simulink model "ASM_sim"  (R2020a)
settings: Solver=ode1  StartTime=0.0  StopTime=70  FixedStep=0.001  RelTol=1e-3
undefined symbols (not defined in the file or in its folder): kd, kp
settings Model: Creator=yshang  LastModifiedBy=jerry
settings DataIOCC: ReturnWorkspaceOutputs=off
settings DebuggingCC: ArithmeticOperatorsInVariantConditions=warning
settings SFSimCC: SimUseLocalCustomCode=off  CustomCodeUndefinedFunction=UseInterfaceOnly
settings RTWCC: RTWUseLocalCustomCode=off
settings CodeAppCC: StateflowObjectComments=on

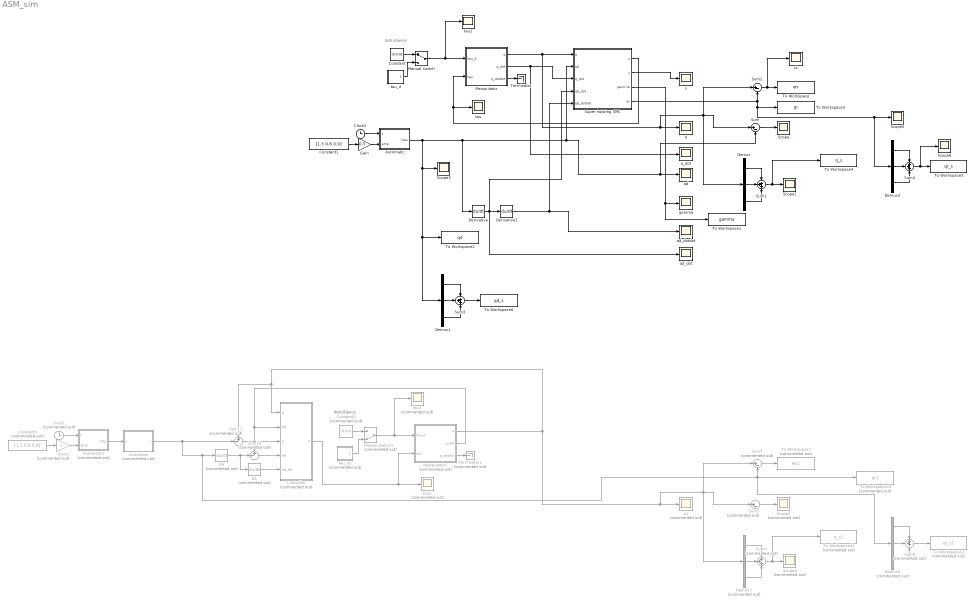
== system ASM_sim ==
  note: disturbance
  note: disturbance
  Automatic : MATLAB Function  TreatAsAtomicUnit=on
  Automatic1 : MATLAB Function  Commented=on  TreatAsAtomicUnit=on
  Clock1 : Clock  Commented=on
  Clock2 : Clock
  Constant : Constant  Value=[0;0;0]
  Constant1 : Constant  Value=[1.5 0.6 0.9]'  SampleTime=0.001
  Constant2 : Constant  Commented=on  Value=[0;0;0]
  Constant3 : Constant  Commented=on  Value=[1.5 0.6 0.9]'  SampleTime=0.001
  Controller : Subsystem  Commented=on
  D4 : Derivative  Commented=on
  D5 : Derivative  Commented=on
  Demux : Demux  Outputs=3
  Demux1 : Demux  Outputs=3
  Demux2 : Demux  Outputs=3
  Demux3 : Demux  Commented=on  Outputs=3
  Demux5 : Demux  Commented=on  Outputs=3
  Derivative : Derivative
  Derivative1 : Derivative
  Gain : Gain  Gain=0.5
  Gain1 : Gain  Commented=on
  Invariance : MATLAB Function  Commented=on  TreatAsAtomicUnit=on
  Manipulator : Subsystem
  Manipulator1 : Subsystem  Commented=on
  Manual Switch : ManualSwitch
  Manual Switch1 : ManualSwitch  Commented=on  CurrentSetting=0
  Scope{,1,3,5..6} (5 alike) : Scope
  Scope2 : Scope  Commented=on
  Scope4 : Scope  Commented=on
  Sum : Sum  Inputs=|+-
  Sum1 : Sum  Inputs=+++
  Sum10 : Sum  Commented=on  Inputs=+-|
  Sum11 : Sum  Commented=on  Inputs=+-|
  Sum2 : Sum  Inputs=|+-
  Sum3 : Sum  Inputs=+++
  Sum4 : Sum  Inputs=+++
  Sum5 : Sum  Commented=on  Inputs=|+-
  Sum6 : Sum  Commented=on  Inputs=+++
  Sum7 : Sum  Commented=on  Inputs=|+-
  Sum9 : Sum  Commented=on  Inputs=+++
  Super twisting SMC : Subsystem
  Terminator : Terminator
  Terminator1 : Terminator  Commented=on
  To Workspace : ToWorkspace  VariableName=err  SampleTime=0.001
  To Workspace1 : ToWorkspace  VariableName=gamma  SampleTime=0.001
  To Workspace10 : ToWorkspace  Commented=on  VariableName=qr1  SampleTime=0.001
  To Workspace11 : ToWorkspace  Commented=on  VariableName=q_s1  SampleTime=0.001
  To Workspace12 : ToWorkspace  Commented=on  VariableName=qr_s1  SampleTime=0.001
  To Workspace2 : ToWorkspace  VariableName=qd  SampleTime=0.001
  To Workspace3 : ToWorkspace  VariableName=qr  SampleTime=0.001
  To Workspace4 : ToWorkspace  VariableName=q_s  SampleTime=0.001
  To Workspace5 : ToWorkspace  VariableName=qr_s  SampleTime=0.001
  To Workspace6 : ToWorkspace  VariableName=qd_s  SampleTime=0.001
  To Workspace7 : ToWorkspace  Commented=on  VariableName=err1  SampleTime=0.001
  gamma : Scope
  q : Scope
  q1 : Scope  Commented=on
  q_dot : Scope
  qd : Scope
  qd_dot : Scope
  qd_dotdot : Scope
  s : Scope
  s1 : Scope
  tau : Scope
  tau1 : Scope
  tau2 : Scope  Commented=on
  tau3 : Scope  Commented=on
  tau_d : Subsystem
  tau_d1 : Subsystem  Commented=on
  wires:
  Manual Switch/1 -> tau1/1, Manipulator/1(tau_d)
  Constant/1 -> Manual Switch/1
  Manipulator/1(q) -> Super twisting SMC/1(q), Sum2/1, Demux/1, Sum/1, q/1
  Manipulator/2(q_dot) -> Super twisting SMC/3(q_dot), q_dot/1
  Super twisting SMC/1(u) -> Manipulator/2(tau), tau/1
  tau_d/1(tau_dist) -> Manual Switch/2
  Super twisting SMC/2(s) -> s/1
  Super twisting SMC/3(gamma) -> To Workspace1/1, gamma/1
  Derivative/1 -> Super twisting SMC/4(qd_dot), qd_dot/1, Derivative1/1
  Manipulator/3(q_dotdot) -> Terminator/1
  Derivative1/1 -> Super twisting SMC/5(qd_dotdot), qd_dotdot/1
  Sum/1 -> Scope/1
  Demux/2 -> Sum1/2
  Demux/1 -> Sum1/1
  Demux/3 -> Sum1/3
  Sum1/1 -> To Workspace4/1, Scope1/1
  Constant1/1 -> Gain/1
  Clock2/1 -> Automatic/1(t)
  Gain/1 -> Automatic/2(amp)
  Sum2/1 -> s1/1, To Workspace/1
  Demux1/2 -> Sum3/2
  Demux1/1 -> Sum3/1
  Automatic/1(Des) -> Demux1/1, To Workspace2/1, Scope3/1, Derivative/1, Super twisting SMC/2(qd), Sum/2, qd/1
  Sum3/1 -> To Workspace6/1
  Demux1/3 -> Sum3/3
  Demux2/2 -> Sum4/2
  Demux2/1 -> Sum4/1
  Super twisting SMC/4(qr) -> Scope5/1, Demux2/1, To Workspace3/1, Sum2/2
  Sum4/1 -> Scope6/1, To Workspace5/1
  Demux2/3 -> Sum4/3
  Sum7/1 -> To Workspace7/1
  Sum6/1 -> To Workspace11/1, Scope4/1
  Demux5/3 -> Sum9/3
  Demux3/1 -> Sum6/1
  Constant2/1 -> Manual Switch1/1
  Invariance/1(y) -> Demux5/1, To Workspace10/1, Sum7/2, D4/1, Sum11/2
  tau_d1/1(tau_dist) -> Manual Switch1/2
  Sum5/1 -> Scope2/1
  Manipulator1/3(q_dotdot) -> Terminator1/1
  Demux5/2 -> Sum9/2
  Controller/1(T) -> Manipulator1/2(tau), tau2/1
  Manual Switch1/1 -> tau3/1, Manipulator1/1(tau_d)
  Demux3/3 -> Sum6/3
  Demux3/2 -> Sum6/2
  Demux5/1 -> Sum9/1
  Sum9/1 -> To Workspace12/1
  Gain1/1 -> Automatic1/2(amp)
  Clock1/1 -> Automatic1/1(t)
  Constant3/1 -> Gain1/1
  Automatic1/1(Des) -> Invariance/1(u)
  Sum11/1 -> Controller/3(e)
  Manipulator1/2(q_dot) -> Controller/2(qd), Sum10/1
  Manipulator1/1(q) -> Sum11/1, Controller/1(q), Sum7/1, Demux3/1, Sum5/1, q1/1
  D4/1 -> D5/1, Sum10/2
  D5/1 -> Controller/5(qd_dd)
  Sum10/1 -> Controller/4(ed)

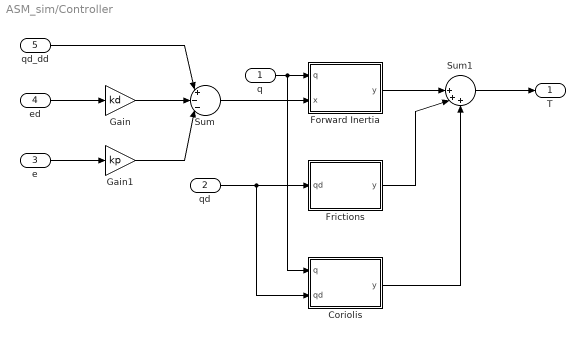
== system ASM_sim/Controller ==
  q : Inport
  qd : Inport  Port=2
  e : Inport  Port=3
  ed : Inport  Port=4
  qd_dd : Inport  Port=5
  Coriolis : MATLAB Function  TreatAsAtomicUnit=on
  Forward Inertia : MATLAB Function  TreatAsAtomicUnit=on
  Frictions : MATLAB Function  TreatAsAtomicUnit=on
  Gain : Gain  Gain=kd
  Gain1 : Gain  Gain=kp
  Sum : Sum  Inputs=|+--|
  Sum1 : Sum  Inputs=||+++
  T : Outport
  wires:
  q/1 -> Coriolis/1(q), Forward Inertia/1(q)
  qd_dd/1 -> Sum/1
  ed/1 -> Gain/1
  Gain/1 -> Sum/2
  e/1 -> Gain1/1
  Gain1/1 -> Sum/3
  Sum/1 -> Forward Inertia/2(x)
  qd/1 -> Coriolis/2(qd), Frictions/1(qd)
  Forward Inertia/1(y) -> Sum1/1
  Frictions/1(y) -> Sum1/2
  Sum1/1 -> T/1
  Coriolis/1(y) -> Sum1/3

== system ASM_sim/Manipulator ==
  tau_d : Inport
  tau : Inport  Port=2
  Integrator : Integrator  InitialCondition=[0;0;0]  ContinuousStateAttributes='velocity'
  Integrator1 : Integrator  InitialCondition=[0;0;0]  ContinuousStateAttributes='position'
  Robot : MATLAB Function  TreatAsAtomicUnit=on
  Sum : Sum  Inputs=|++
  q : Outport  VectorParamsAs1DForOutWhenUnconnected=off
  q_dot : Outport  Port=2  VectorParamsAs1DForOutWhenUnconnected=off
  q_dotdot : Outport  Port=3  VectorParamsAs1DForOutWhenUnconnected=off
  wires:
  Integrator1/1 -> Robot/2(q), q/1
  Robot/1(qdd) -> q_dotdot/1, Integrator/1
  Integrator/1 -> q_dot/1, Robot/3(qd), Integrator1/1
  Sum/1 -> Robot/1(T)
  tau_d/1 -> Sum/1
  tau/1 -> Sum/2

== system ASM_sim/Manipulator1 ==
  tau_d : Inport
  tau : Inport  Port=2
  Integrator : Integrator  InitialCondition=[0;0;0]  ContinuousStateAttributes='velocity'
  Integrator1 : Integrator  InitialCondition=[0;0;0]  ContinuousStateAttributes='position'
  Robot : MATLAB Function  TreatAsAtomicUnit=on
  Sum : Sum  Inputs=|++
  q : Outport  VectorParamsAs1DForOutWhenUnconnected=off
  q_dot : Outport  Port=2  VectorParamsAs1DForOutWhenUnconnected=off
  q_dotdot : Outport  Port=3  VectorParamsAs1DForOutWhenUnconnected=off
  wires:
  Integrator1/1 -> Robot/2(q), q/1
  Robot/1(qdd) -> q_dotdot/1, Integrator/1
  Integrator/1 -> q_dot/1, Robot/3(qd), Integrator1/1
  Sum/1 -> Robot/1(T)
  tau_d/1 -> Sum/1
  tau/1 -> Sum/2

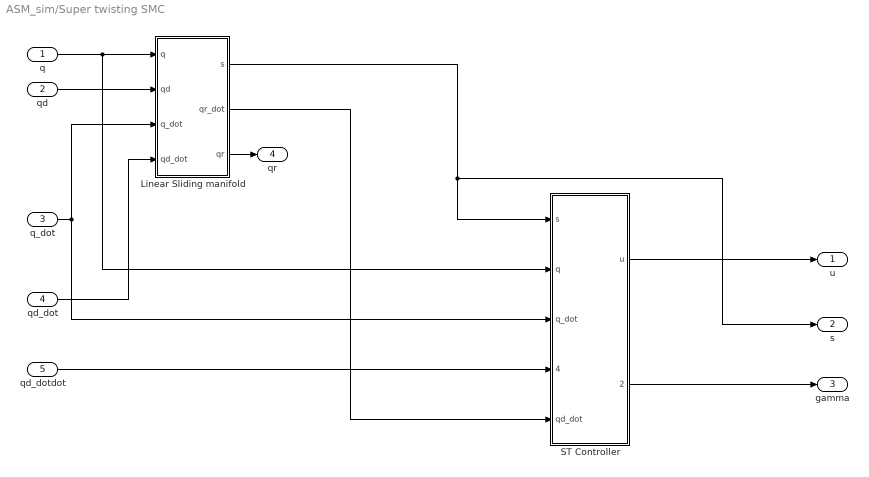
== system ASM_sim/Super twisting SMC ==
  q : Inport
  qd : Inport  Port=2
  q_dot : Inport  Port=3
  qd_dot : Inport  Port=4
  qd_dotdot : Inport  Port=5
  Linear Sliding manifold : Subsystem
  ST Controller : Subsystem
  u : Outport  VectorParamsAs1DForOutWhenUnconnected=off
  s : Outport  Port=2  VectorParamsAs1DForOutWhenUnconnected=off
  gamma : Outport  Port=3  VectorParamsAs1DForOutWhenUnconnected=off
  qr : Outport  Port=4  VectorParamsAs1DForOutWhenUnconnected=off
  wires:
  q/1 -> Linear Sliding manifold/1(q), ST Controller/2(q)
  q_dot/1 -> Linear Sliding manifold/3(q_dot), ST Controller/3(q_dot)
  Linear Sliding manifold/1(s) -> s/1, ST Controller/1(s)
  qd/1 -> Linear Sliding manifold/2(qd)
  ST Controller/1(u) -> u/1
  ST Controller/2(gamma) -> gamma/1
  qd_dot/1 -> Linear Sliding manifold/4(qd_dot)
  qd_dotdot/1 -> ST Controller/4(qd_dotdot)
  Linear Sliding manifold/2(qr_dot) -> ST Controller/5("qd_dot ")
  Linear Sliding manifold/3(qr) -> qr/1

== system ASM_sim/tau_d ==
  Mux1 : Mux  Inputs=3
  Sine Wave3 : Sin  Amplitude=0.3  Frequency=2  SampleTime=0
  Sine Wave4 : Sin  Amplitude=0.2  Frequency=4  SampleTime=0
  Sine Wave5 : Sin  Amplitude=0.1  Frequency=3  SampleTime=0
  tau_dist : Outport  VectorParamsAs1DForOutWhenUnconnected=off
  wires:
  Sine Wave4/1 -> Mux1/2
  Mux1/1 -> tau_dist/1
  Sine Wave3/1 -> Mux1/1
  Sine Wave5/1 -> Mux1/3

== system ASM_sim/tau_d1 ==
  Mux1 : Mux  Inputs=3
  Sine Wave3 : Sin  Amplitude=0.3  Frequency=2  SampleTime=0
  Sine Wave4 : Sin  Amplitude=0.2  Frequency=4  SampleTime=0
  Sine Wave5 : Sin  Amplitude=0.1  Frequency=3  SampleTime=0
  tau_dist : Outport  VectorParamsAs1DForOutWhenUnconnected=off
  wires:
  Sine Wave4/1 -> Mux1/2
  Mux1/1 -> tau_dist/1
  Sine Wave3/1 -> Mux1/1
  Sine Wave5/1 -> Mux1/3

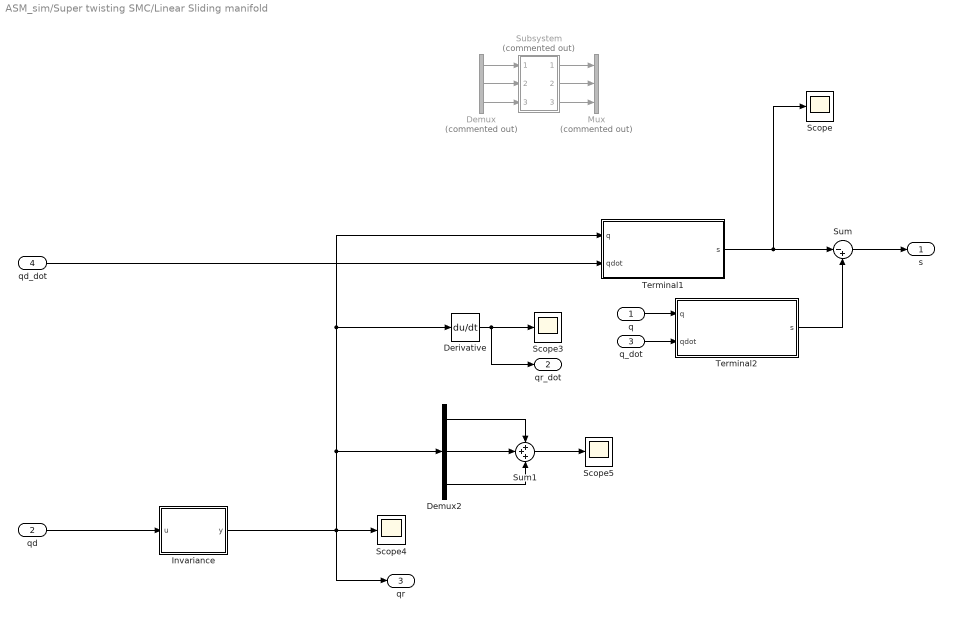
== system ASM_sim/Super twisting SMC/Linear Sliding manifold ==
  q : Inport
  qd : Inport  Port=2
  q_dot : Inport  Port=3
  qd_dot : Inport  Port=4
  Demux : Demux  Commented=on  Outputs=3
  Demux2 : Demux  Outputs=3
  Derivative : Derivative
  Invariance : MATLAB Function  TreatAsAtomicUnit=on
  Mux : Mux  Commented=on  Inputs=3
  Scope{,3..5} (4 alike) : Scope
  Subsystem : Subsystem  Commented=on
  Sum : Sum  Inputs=|-+
  Sum1 : Sum  Inputs=+++
  Terminal1 : Subsystem
  Terminal2 : Subsystem
  s : Outport  VectorParamsAs1DForOutWhenUnconnected=off
  qr_dot : Outport  Port=2  VectorParamsAs1DForOutWhenUnconnected=off
  qr : Outport  Port=3  VectorParamsAs1DForOutWhenUnconnected=off
  wires:
  q/1 -> Terminal2/1(q)
  q_dot/1 -> Terminal2/2(qdot)
  Terminal2/1(s) -> Sum/2
  Sum/1 -> s/1
  Demux2/3 -> Sum1/3
  qd/1 -> Invariance/1(u)
  Derivative/1 -> qr_dot/1, Scope3/1
  Demux2/2 -> Sum1/2
  Sum1/1 -> Scope5/1
  Demux2/1 -> Sum1/1
  Terminal1/1(s) -> Scope/1, Sum/1
  qd_dot/1 -> Terminal1/2(qdot)
  Invariance/1(y) -> qr/1, Demux2/1, Terminal1/1(q), Derivative/1, Scope4/1
  Demux/2 -> Subsystem/2(In2)
  Subsystem/3(Out3) -> Mux/3
  Demux/1 -> Subsystem/1(In1)
  Subsystem/1(Out1) -> Mux/1
  Demux/3 -> Subsystem/3(In3)
  Subsystem/2(Out2) -> Mux/2

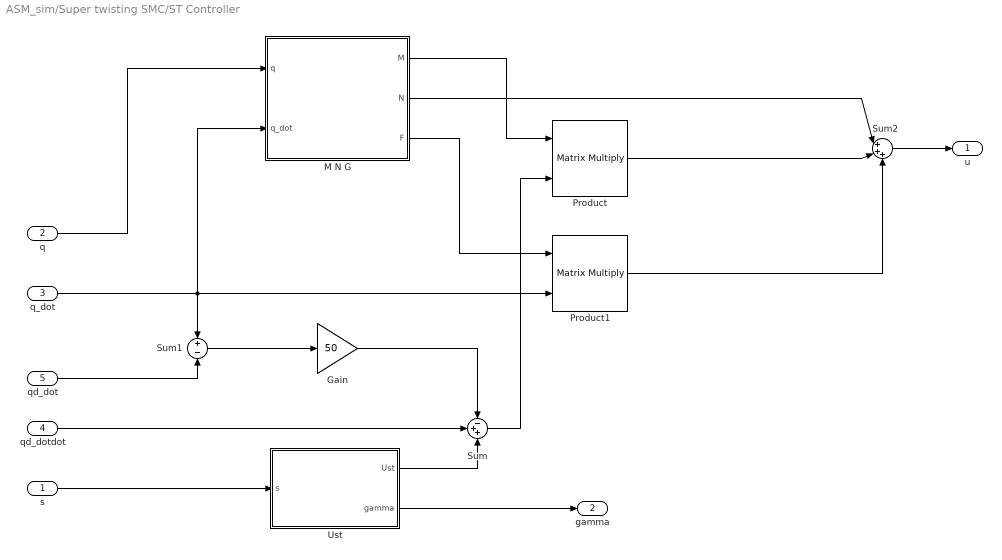
== system ASM_sim/Super twisting SMC/ST Controller ==
  s : Inport
  q : Inport  Port=2
  q_dot : Inport  Port=3
  qd_dotdot : Inport  Port=4
  "qd_dot " : Inport  Port=5
  Gain : Gain  Gain=50
  M N G : MATLAB Function  TreatAsAtomicUnit=on
  Product : Product  Multiplication=Matrix(*)
  Product1 : Product  Multiplication=Matrix(*)
  Sum : Sum  Inputs=-++
  Sum1 : Sum  Inputs=+|-
  Sum2 : Sum  Inputs=|+++
  Ust : Subsystem
  u : Outport  VectorParamsAs1DForOutWhenUnconnected=off
  gamma : Outport  Port=2  VectorParamsAs1DForOutWhenUnconnected=off
  wires:
  s/1 -> Ust/1(s)
  Ust/2(gamma) -> gamma/1
  Sum/1 -> Product/2
  Ust/1(Ust) -> Sum/3
  M N G/3(F) -> Product1/1
  M N G/1(M) -> Product/1
  q/1 -> M N G/1(q)
  q_dot/1 -> M N G/2(q_dot), Product1/2, Sum1/1
  Product1/1 -> Sum2/3
  Sum2/1 -> u/1
  "qd_dot "/1 -> Sum1/2
  Sum1/1 -> Gain/1
  qd_dotdot/1 -> Sum/2
  Gain/1 -> Sum/1
  M N G/2(N) -> Sum2/1
  Product/1 -> Sum2/2

== system ASM_sim/Super twisting SMC/Linear Sliding manifold/Subsystem ==
  In1 : Inport
  In2 : Inport  Port=2
  In3 : Inport  Port=3
  Transfer Fcn : TransferFcn  Denominator=[0.01 1]
  Transfer Fcn1 : TransferFcn  Denominator=[0.01 1]
  Transfer Fcn2 : TransferFcn  Denominator=[0.01 1]
  Out1 : Outport
  Out2 : Outport  Port=2
  Out3 : Outport  Port=3
  wires:
  Transfer Fcn/1 -> Out1/1
  Transfer Fcn1/1 -> Out2/1
  In2/1 -> Transfer Fcn1/1
  In1/1 -> Transfer Fcn/1
  Transfer Fcn2/1 -> Out3/1
  In3/1 -> Transfer Fcn2/1

== system ASM_sim/Super twisting SMC/Linear Sliding manifold/Terminal1 ==
  q : Inport
  qdot : Inport  Port=2
  Gain1 : Gain  Gain=50
  Sum5 : Sum  Inputs=|++
  s : Outport  VectorParamsAs1DForOutWhenUnconnected=off
  wires:
  q/1 -> Gain1/1
  Sum5/1 -> s/1
  Gain1/1 -> Sum5/1
  qdot/1 -> Sum5/2

== system ASM_sim/Super twisting SMC/Linear Sliding manifold/Terminal2 ==
  q : Inport
  qdot : Inport  Port=2
  Gain1 : Gain  Gain=50
  Sum5 : Sum  Inputs=|++
  s : Outport  VectorParamsAs1DForOutWhenUnconnected=off
  wires:
  q/1 -> Gain1/1
  Sum5/1 -> s/1
  Gain1/1 -> Sum5/1
  qdot/1 -> Sum5/2

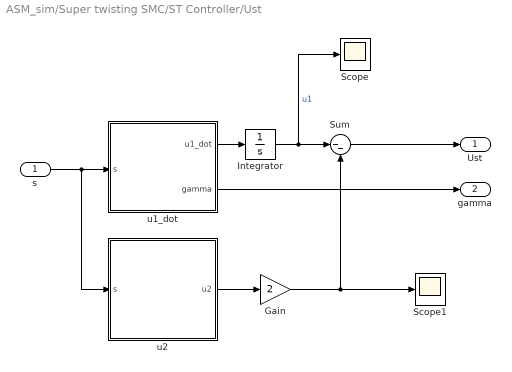
== system ASM_sim/Super twisting SMC/ST Controller/Ust ==
  s : Inport
  Gain : Gain  Gain=2
  Integrator : Integrator
  Scope : Scope
  Scope1 : Scope
  Sum : Sum  Inputs=|--
  u1_dot : Subsystem
  u2 : Subsystem
  Ust : Outport  VectorParamsAs1DForOutWhenUnconnected=off
  gamma : Outport  Port=2  VectorParamsAs1DForOutWhenUnconnected=off
  wires:
  s/1 -> u2/1(s), u1_dot/1(s)
  u1_dot/1(u1_dot) -> Integrator/1
  Integrator/1 -> Sum/1, Scope/1  "u1"
  u2/1(u2) -> Gain/1
  Sum/1 -> Ust/1
  u1_dot/2(gamma) -> gamma/1
  Gain/1 -> Scope1/1, Sum/2

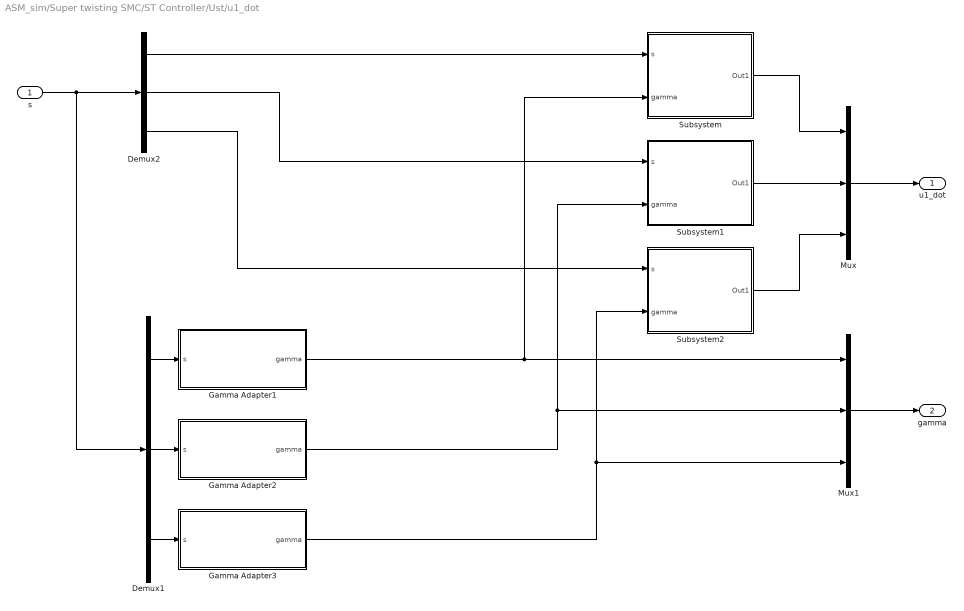
== system ASM_sim/Super twisting SMC/ST Controller/Ust/u1_dot ==
  s : Inport
  Demux1 : Demux  Outputs=3
  Demux2 : Demux  Outputs=3
  Gamma Adapter1 : Subsystem
  Gamma Adapter2 : Subsystem
  Gamma Adapter3 : Subsystem
  Mux : Mux  Inputs=3
  Mux1 : Mux  Inputs=3
  Subsystem : Subsystem
  Subsystem1 : Subsystem
  Subsystem2 : Subsystem
  u1_dot : Outport  VectorParamsAs1DForOutWhenUnconnected=off
  gamma : Outport  Port=2  VectorParamsAs1DForOutWhenUnconnected=off
  wires:
  Mux/1 -> u1_dot/1
  s/1 -> Demux1/1, Demux2/1
  Demux2/1 -> Subsystem/1(s)
  Demux2/2 -> Subsystem1/1(s)
  Subsystem1/1(Out1) -> Mux/2
  Subsystem/1(Out1) -> Mux/1
  Subsystem2/1(Out1) -> Mux/3
  Demux2/3 -> Subsystem2/1(s)
  Demux1/1 -> Gamma Adapter1/1(s)
  Demux1/3 -> Gamma Adapter3/1(s)
  Demux1/2 -> Gamma Adapter2/1(s)
  Mux1/1 -> gamma/1
  Gamma Adapter1/1(gamma) -> Subsystem/2(gamma), Mux1/1
  Gamma Adapter2/1(gamma) -> Subsystem1/2(gamma), Mux1/2
  Gamma Adapter3/1(gamma) -> Subsystem2/2(gamma), Mux1/3

== system ASM_sim/Super twisting SMC/ST Controller/Ust/u2 ==
  s : Inport
  Demux : Demux  Outputs=3
  Mux : Mux  Inputs=3
  Subsystem : Subsystem
  Subsystem1 : Subsystem
  Subsystem3 : Subsystem
  u2 : Outport  VectorParamsAs1DForOutWhenUnconnected=off
  wires:
  Mux/1 -> u2/1
  s/1 -> Demux/1
  Demux/1 -> Subsystem/1(In1)
  Subsystem/1(Out1) -> Mux/1
  Demux/3 -> Subsystem3/1(In1)
  Demux/2 -> Subsystem1/1(In1)
  Subsystem1/1(Out1) -> Mux/2
  Subsystem3/1(Out1) -> Mux/3

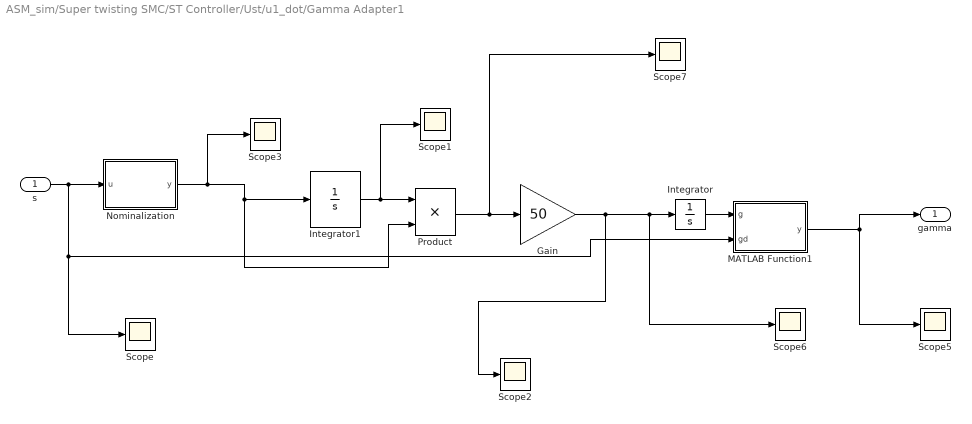
== system ASM_sim/Super twisting SMC/ST Controller/Ust/u1_dot/Gamma Adapter1 ==
  s : Inport
  Gain : Gain  Gain=50
  Integrator : Integrator
  Integrator1 : Integrator
  MATLAB Function1 : MATLAB Function  TreatAsAtomicUnit=on
  Nominalization : MATLAB Function  TreatAsAtomicUnit=on
  Product : Product
  Scope{,1..3,5..7} (7 alike) : Scope
  gamma : Outport  VectorParamsAs1DForOutWhenUnconnected=off
  wires:
  MATLAB Function1/1(y) -> gamma/1, Scope5/1
  Integrator1/1 -> Product/1, Scope1/1
  s/1 -> Scope/1, MATLAB Function1/2(gd), Nominalization/1(u)
  Nominalization/1(y) -> Integrator1/1, Product/2, Scope3/1
  Product/1 -> Gain/1, Scope7/1
  Gain/1 -> Scope6/1, Integrator/1, Scope2/1
  Integrator/1 -> MATLAB Function1/1(g)

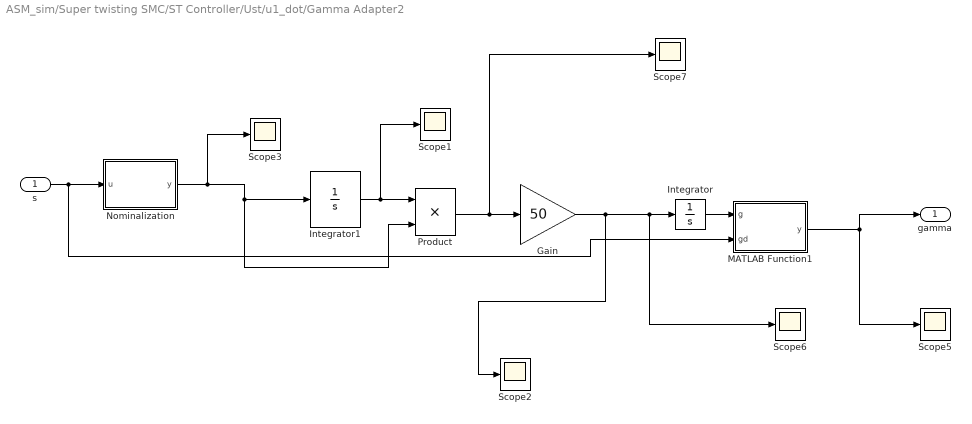
== system ASM_sim/Super twisting SMC/ST Controller/Ust/u1_dot/Gamma Adapter2 ==
  s : Inport
  Gain : Gain  Gain=50
  Integrator : Integrator
  Integrator1 : Integrator
  MATLAB Function1 : MATLAB Function  TreatAsAtomicUnit=on
  Nominalization : MATLAB Function  TreatAsAtomicUnit=on
  Product : Product
  Scope{1..3,5..7} (6 alike) : Scope
  gamma : Outport  VectorParamsAs1DForOutWhenUnconnected=off
  wires:
  Integrator/1 -> MATLAB Function1/1(g)
  Gain/1 -> Scope2/1, Integrator/1, Scope6/1
  Product/1 -> Scope7/1, Gain/1
  Nominalization/1(y) -> Scope3/1, Product/2, Integrator1/1
  s/1 -> Nominalization/1(u), MATLAB Function1/2(gd)
  Integrator1/1 -> Scope1/1, Product/1
  MATLAB Function1/1(y) -> Scope5/1, gamma/1

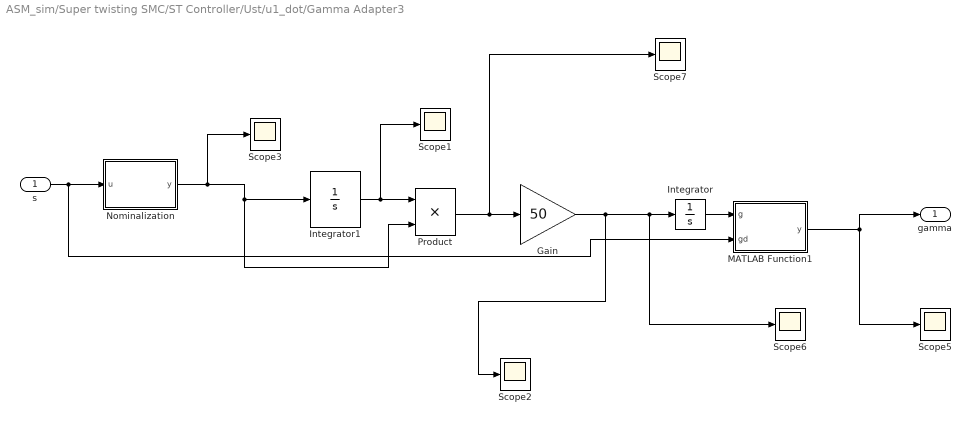
== system ASM_sim/Super twisting SMC/ST Controller/Ust/u1_dot/Gamma Adapter3 ==
  s : Inport
  Gain : Gain  Gain=50
  Integrator : Integrator
  Integrator1 : Integrator
  MATLAB Function1 : MATLAB Function  TreatAsAtomicUnit=on
  Nominalization : MATLAB Function  TreatAsAtomicUnit=on
  Product : Product
  Scope{1..3,5..7} (6 alike) : Scope
  gamma : Outport  VectorParamsAs1DForOutWhenUnconnected=off
  wires:
  MATLAB Function1/1(y) -> gamma/1, Scope5/1
  Integrator1/1 -> Product/1, Scope1/1
  s/1 -> MATLAB Function1/2(gd), Nominalization/1(u)
  Nominalization/1(y) -> Integrator1/1, Product/2, Scope3/1
  Product/1 -> Gain/1, Scope7/1
  Gain/1 -> Scope6/1, Integrator/1, Scope2/1
  Integrator/1 -> MATLAB Function1/1(g)

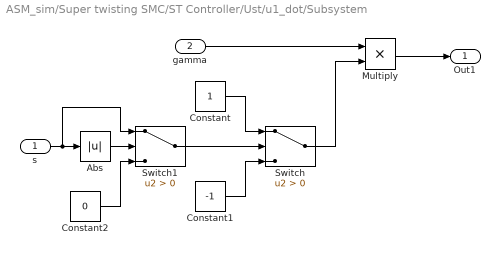
== system ASM_sim/Super twisting SMC/ST Controller/Ust/u1_dot/Subsystem ==
  s : Inport
  gamma : Inport  Port=2
  Abs : Abs
  Constant : Constant
  Constant1 : Constant  Value=-1
  Constant2 : Constant  Value=0
  Multiply : Product
  Switch : Switch  Criteria=u2 > Threshold
  Switch1 : Switch  Criteria=u2 > Threshold
  Out1 : Outport  VectorParamsAs1DForOutWhenUnconnected=off
  wires:
  Switch/1 -> Multiply/2
  s/1 -> Switch1/1, Abs/1
  gamma/1 -> Multiply/1
  Multiply/1 -> Out1/1
  Constant/1 -> Switch/1
  Constant1/1 -> Switch/3
  Abs/1 -> Switch1/2
  Constant2/1 -> Switch1/3
  Switch1/1 -> Switch/2

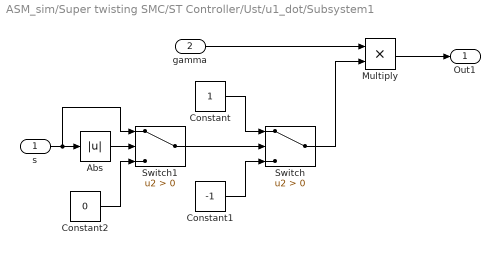
== system ASM_sim/Super twisting SMC/ST Controller/Ust/u1_dot/Subsystem1 ==
  s : Inport
  gamma : Inport  Port=2
  Abs : Abs
  Constant : Constant
  Constant1 : Constant  Value=-1
  Constant2 : Constant  Value=0
  Multiply : Product
  Switch : Switch  Criteria=u2 > Threshold
  Switch1 : Switch  Criteria=u2 > Threshold
  Out1 : Outport  VectorParamsAs1DForOutWhenUnconnected=off
  wires:
  Switch1/1 -> Switch/2
  Constant2/1 -> Switch1/3
  Abs/1 -> Switch1/2
  Constant1/1 -> Switch/3
  Constant/1 -> Switch/1
  Multiply/1 -> Out1/1
  gamma/1 -> Multiply/1
  s/1 -> Abs/1, Switch1/1
  Switch/1 -> Multiply/2

== system ASM_sim/Super twisting SMC/ST Controller/Ust/u1_dot/Subsystem2 ==
  s : Inport
  gamma : Inport  Port=2
  Abs : Abs
  Constant : Constant
  Constant1 : Constant  Value=-1
  Constant2 : Constant  Value=0
  Multiply : Product
  Switch : Switch  Criteria=u2 > Threshold
  Switch1 : Switch  Criteria=u2 > Threshold
  Out1 : Outport  VectorParamsAs1DForOutWhenUnconnected=off
  wires:
  Switch/1 -> Multiply/2
  s/1 -> Switch1/1, Abs/1
  gamma/1 -> Multiply/1
  Multiply/1 -> Out1/1
  Constant/1 -> Switch/1
  Constant1/1 -> Switch/3
  Abs/1 -> Switch1/2
  Constant2/1 -> Switch1/3
  Switch1/1 -> Switch/2

== system ASM_sim/Super twisting SMC/ST Controller/Ust/u2/Subsystem ==
  In1 : Inport
  Abs : Abs
  Abs1 : Abs
  Gain : Gain  Gain=-1
  Scope : Scope
  Scope1 : Scope
  Sqrt1 : Sqrt  SaturateOnIntegerOverflow=on
  Sqrt2 : Sqrt  SaturateOnIntegerOverflow=on
  Switch : Switch  Criteria=u2 > Threshold
  Out1 : Outport  VectorParamsAs1DForOutWhenUnconnected=off
  wires:
  In1/1 -> Scope/1, Abs/1, Switch/2, Abs1/1
  Switch/1 -> Out1/1, Scope1/1
  Sqrt1/1 -> Switch/1
  Sqrt2/1 -> Gain/1
  Abs/1 -> Sqrt1/1
  Abs1/1 -> Sqrt2/1
  Gain/1 -> Switch/3

== system ASM_sim/Super twisting SMC/ST Controller/Ust/u2/Subsystem1 ==
  In1 : Inport
  Abs : Abs
  Abs1 : Abs
  Gain : Gain  Gain=-1
  Scope : Scope
  Scope1 : Scope
  Sqrt1 : Sqrt  SaturateOnIntegerOverflow=on
  Sqrt2 : Sqrt  SaturateOnIntegerOverflow=on
  Switch : Switch  Criteria=u2 > Threshold
  Out1 : Outport  VectorParamsAs1DForOutWhenUnconnected=off
  wires:
  Gain/1 -> Switch/3
  Abs1/1 -> Sqrt2/1
  Abs/1 -> Sqrt1/1
  Sqrt2/1 -> Gain/1
  Sqrt1/1 -> Switch/1
  Switch/1 -> Scope1/1, Out1/1
  In1/1 -> Abs1/1, Switch/2, Abs/1, Scope/1

== system ASM_sim/Super twisting SMC/ST Controller/Ust/u2/Subsystem3 ==
  In1 : Inport
  Abs : Abs
  Abs1 : Abs
  Gain : Gain  Gain=-1
  Scope : Scope
  Scope1 : Scope
  Sqrt1 : Sqrt  SaturateOnIntegerOverflow=on
  Sqrt2 : Sqrt  SaturateOnIntegerOverflow=on
  Switch : Switch  Criteria=u2 > Threshold
  Out1 : Outport  VectorParamsAs1DForOutWhenUnconnected=off
  wires:
  In1/1 -> Scope/1, Abs/1, Switch/2, Abs1/1
  Switch/1 -> Out1/1, Scope1/1
  Sqrt1/1 -> Switch/1
  Sqrt2/1 -> Gain/1
  Abs/1 -> Sqrt1/1
  Abs1/1 -> Sqrt2/1
  Gain/1 -> Switch/3

== matlab function ASM_sim/Invariance ==
  data: u input; y output
function y = fcn(u)


A1 = [1,1,1];
b1 = 2.9;
A2 = [-1,-1,-1];
b2 = 2.9;


if A1*u>b1
y = A1'/(A1*A1')*(b1-A1*u)+u;
elseif A2*u>b2
y = A2'/(A2*A2')*(b2-A2*u)+u;
else
y=u;
end

== matlab function ASM_sim/Controller/Coriolis ==
  data: q input; y output; qd input
function y = fcn(q,qd)
%#codegen

% cos and sine
% c2=cos(q(2));
% c3=cos(q(3));
% c23=cos(q(2)+q(3));
s2=sin(q(2));
s3=sin(q(3));
s23=sin(q(2)+q(3));
% N-components
n11 = -.1742*s2*qd(2)^2-0.04047*s23*qd(2)^2-.02809*s3*qd(3)^2-.04047*s23*qd(3)^2-0.3484*s2*qd(1)*qd(2)-.08094*s23*qd(1)*qd(2);
n12 = -0.05619*s3*qd(1)*qd(3)-.08094*s23*qd(1)*qd(3)-.05619*s3*qd(2)*qd(3)-.08094*s23*qd(2)*qd(3);
n2 = .1742*s2*qd(1)^2+.04047*s23*qd(1)^2-.02809*s3*qd(3)^2-0.0561*s3*qd(1)*qd(3)-0.05619*s3*qd(2)*qd(3);
n3 = 0.02809*s3*qd(1)^2+.02809*s3*qd(2)^2+.04047*s23*qd(1)^2+.05619*s3*qd(1)*qd(2);
% N matrix
N = [n11+n12;
     n2;
     n3];

y = N;

== matlab function ASM_sim/Controller/Forward Inertia ==
  data: q input; y output; x input
function y = fcn(q,x)


% cos
c2 = cos(q(2));
c3 = cos(q(3));
c23 = cos(q(2)+q(3));
% M-components
m11 = 1.0425+0.08094*c23+0.3484*c2+.0561*c3;
m12 = 0.4398+.04047*c23+.1742*c2+.0561*c3;
m13 = .1788+.04047*c23+.02809*c3;
m22 = .4398+.0519*c3;
m23 = .1788+.02809*c3;
m33 = .1788; 

M = [m11 m12 m13;
     m12 m22 m23;
     m13 m23 m33];

y = M*x;

== matlab function ASM_sim/Controller/Frictions ==
  data: qd input; y output
function y = fcn(qd)
%#codegen

F=[2.6e-4 0 0;
   0 2.6e-4 0;
   0 0 2.6e-4];

y = F*qd;

== matlab function ASM_sim/Automatic ==
  data: t input size=1; Des output size=3; amp input size=3
function Des = fcn(t,amp)

ph = [3 8 5]';
Des = [0 0 0]';

if (t >= 11) && (t < 59)
    Des(1) = -2*cos(2*pi/16*(t-ph(1)))*amp(1);
elseif (t >= 3) && (t < 67)
    Des(1) = (1-cos(2*pi/16*(t-ph(1))))*amp(1);
else
    Des(1) = 0;
end

if (t >= 11+5) && (t < 59+5)
    Des(2) = -2*cos(2*pi/16*(t-ph(2)))*amp(2);
elseif (t >= 3+5) && (t < 67+5)
    Des(2) = (1-cos(2*pi/16*(t-ph(2))))*amp(2);
else
    Des(2) = 0;
end

if (t >= 11+2) && (t < 59+2)
    Des(3) = -2*cos(2*pi/16*(t-ph(3)))*amp(3);
elseif (t >= 3+2) && (t < 67+2)
    Des(3) = (1-cos(2*pi/16*(t-ph(3))))*amp(3);
else
    Des(3) = 0;
end

== matlab function ASM_sim/Super twisting SMC/ST Controller/Ust/u1_dot/Gamma Adapter2/MATLAB Function1 ==
  settings: updateMethod=DISCRETE
  data: g input; y output; gd input
function y = fcn(g, gd)
persistent temp;

if isempty(temp)
    temp = 0;
end

if abs(gd) < 0.2
    temp = 0.99999*temp;
else
    temp = g;
end

y=temp;

== matlab function ASM_sim/Super twisting SMC/ST Controller/Ust/u1_dot/Gamma Adapter2/Nominalization ==
  data: u input; y output
function y = fcn(u)

y = u/(norm(u,2)+0.02);

== matlab function ASM_sim/Manipulator/Robot ==
  data: T input; qdd output; q input; qd input
function qdd = fcn(T,q,qd)
%#codegen

% cos and sine
c2 = cos(q(2));
c3 = cos(q(3));
c23 = cos(q(2)+q(3));
s2 = sin(q(2));
s3 = sin(q(3));
s23 = sin(q(2)+q(3));
% M-components
m11 = 1.0425+0.08094*c23+0.3484*c2+.0561*c3;
m12 = 0.4398+.04047*c23+.1742*c2+.0561*c3;
m13 = .1788+.04047*c23+.02809*c3;
m22 = .4398+.0519*c3;
m23 = .1788+.02809*c3;
m33 = .1788;
% Mass-Inertia matrix
M = [m11 m12 m13;
     m12 m22 m23;
     m13 m23 m33];
% N-components
n11 = -.1742*s2*qd(2)^2-0.04047*s23*qd(2)^2-.02809*s3*qd(3)^2-.04047*s23*qd(3)^2-0.3484*s2*qd(1)*qd(2)-.08094*s23*qd(1)*qd(2);
n12 = -0.05619*s3*qd(1)*qd(3)-.08094*s23*qd(1)*qd(3)-.05619*s3*qd(2)*qd(3)-.08094*s23*qd(2)*qd(3);
n2 = .1742*s2*qd(1)^2+.04047*s23*qd(1)^2-.02809*s3*qd(3)^2-0.0561*s3*qd(1)*qd(3)-0.05619*s3*qd(2)*qd(3);
n3 = 0.02809*s3*qd(1)^2+.02809*s3*qd(2)^2+.04047*s23*qd(1)^2+.05619*s3*qd(1)*qd(2);
% N matrix
N = [n11+n12;
     n2;
     n3];
% Friction coefficients
F = [2.6e-4 0 0;
     0 2.6e-4 0; 
     0 0 2.6e-4];

qdd=M\(T-N-F*qd);

== matlab function ASM_sim/Super twisting SMC/ST Controller/Ust/u1_dot/Gamma Adapter1/Nominalization ==
  data: u input; y output
function y = fcn(u)

y = u/(norm(u,2)+0.02);

== matlab function ASM_sim/Super twisting SMC/ST Controller/Ust/u1_dot/Gamma Adapter3/MATLAB Function1 ==
  settings: updateMethod=DISCRETE
  data: g input; y output; gd input
function y = fcn(g, gd)
persistent temp;

if isempty(temp)
    temp = 0;
end

if abs(gd) < 0.2
    temp = 0.99999*temp;
else
    temp = g;
end

y=temp;

== matlab function ASM_sim/Super twisting SMC/ST Controller/Ust/u1_dot/Gamma Adapter3/Nominalization ==
  data: u input; y output
function y = fcn(u)

y = u/(norm(u,2)+0.02);

== matlab function ASM_sim/Super twisting SMC/ST Controller/M N G ==
  data: q input; M output; N output; F output; q_dot input
function [M,N,F] = fcn(q,q_dot)

% cos and sine
c2 = cos(q(2));
c3 = cos(q(3));
c23 = cos(q(2)+q(3));
s2 = sin(q(2));
s3 = sin(q(3));
s23 = sin(q(2)+q(3));
% M-components
m11 = 1.0425+0.08094*c23+0.3484*c2+.0561*c3;
m12 = 0.4398+.04047*c23+.1742*c2+.0561*c3;
m13 = .1788+.04047*c23+.02809*c3;
m22 = .4398+.0519*c3;
m23 = .1788+.02809*c3;
m33 = .1788;
% Mass-Inertia matrix
% M = [m11 m12 m13;
%     m12 m22 m23;
%     m13 m23 m33];
     
%M = [1 0 0;
%     0 1 0;
%     0 0 1];
 
 M = 0.5*[1.6 0 0;
     0 1 0;
     0 0 0.7];
 
% N-components
n11 = -.1742*s2*q_dot(2)^2-0.04047*s23*q_dot(2)^2-.02809*s3*q_dot(3)^2-.04047*s23*q_dot(3)^2-0.3484*s2*q_dot(1)*q_dot(2)-.08094*s23*q_dot(1)*q_dot(2);
n12 = -0.05619*s3*q_dot(1)*q_dot(3)-.08094*s23*q_dot(1)*q_dot(3)-.05619*s3*q_dot(2)*q_dot(3)-.08094*s23*q_dot(2)*q_dot(3);
n2 = .1742*s2*q_dot(1)^2+.04047*s23*q_dot(1)^2-.02809*s3*q_dot(3)^2-0.0561*s3*q_dot(1)*q_dot(3)-0.05619*s3*q_dot(2)*q_dot(3);
n3 = 0.02809*s3*q_dot(1)^2+.02809*s3*q_dot(2)^2+.04047*s23*q_dot(1)^2+.05619*s3*q_dot(1)*q_dot(2);
% N matrix
N = [n11+n12;
     n2;
     n3];
% Friction coefficients
F = [2.6e-4 0 0;
      0 2.6e-4 0; 
      0 0 2.6e-4];
% gravity
% G=[0;0;0];

== matlab function ASM_sim/Automatic1 ==
  data: t input size=1; Des output size=3; amp input size=3
function Des = fcn(t,amp)

if (t >= 11) && (t < 59)
    Des = -2*cos(2*pi/16*(t-3))*amp;
elseif (t >= 3) && (t < 67)
    Des = (1-cos(2*pi/16*(t-3)))*amp;
else
    Des = [0 0 0]';
end

== matlab function ASM_sim/Manipulator1/Robot ==
  data: T input; qdd output; q input; qd input
function qdd = fcn(T,q,qd)
%#codegen

% cos and sine
c2 = cos(q(2));
c3 = cos(q(3));
c23 = cos(q(2)+q(3));
s2 = sin(q(2));
s3 = sin(q(3));
s23 = sin(q(2)+q(3));
% M-components
m11 = 1.0425+0.08094*c23+0.3484*c2+.0561*c3;
m12 = 0.4398+.04047*c23+.1742*c2+.0561*c3;
m13 = .1788+.04047*c23+.02809*c3;
m22 = .4398+.0519*c3;
m23 = .1788+.02809*c3;
m33 = .1788;
% Mass-Inertia matrix
M = [m11 m12 m13;
     m12 m22 m23;
     m13 m23 m33];
% N-components
n11 = -.1742*s2*qd(2)^2-0.04047*s23*qd(2)^2-.02809*s3*qd(3)^2-.04047*s23*qd(3)^2-0.3484*s2*qd(1)*qd(2)-.08094*s23*qd(1)*qd(2);
n12 = -0.05619*s3*qd(1)*qd(3)-.08094*s23*qd(1)*qd(3)-.05619*s3*qd(2)*qd(3)-.08094*s23*qd(2)*qd(3);
n2 = .1742*s2*qd(1)^2+.04047*s23*qd(1)^2-.02809*s3*qd(3)^2-0.0561*s3*qd(1)*qd(3)-0.05619*s3*qd(2)*qd(3);
n3 = 0.02809*s3*qd(1)^2+.02809*s3*qd(2)^2+.04047*s23*qd(1)^2+.05619*s3*qd(1)*qd(2);
% N matrix
N = [n11+n12;
     n2;
     n3];
% Friction coefficients
F = [2.6e-4 0 0;
     0 2.6e-4 0; 
     0 0 2.6e-4];

qdd=M\(T-N-F*qd);

== matlab function ASM_sim/Super twisting SMC/Linear Sliding manifold/Invariance ==
  data: u input; y output
function y = fcn(u)


A1 = [1,1,1];
b1 = 1.4;
A2 = [-1,-1,-1];
b2 = 1.4;


if A1*u>b1
y = A1'/(A1*A1')*(b1-A1*u)+u;
elseif A2*u>b2
y = A2'/(A2*A2')*(b2-A2*u)+u;
else
y=u;
end

== matlab function ASM_sim/Super twisting SMC/ST Controller/Ust/u1_dot/Gamma Adapter1/MATLAB Function1 ==
  settings: updateMethod=DISCRETE
  data: g input; y output; gd input
function y = fcn(g, gd)
persistent temp;

if isempty(temp)
    temp = 0;
end

if abs(gd) < 0.2
    temp = 0.99999*temp;
else
    temp = g;
end

y=temp;
